simulink library "Lib_PF_SwitchDC_TMATS"  (R2017a)
settings: Solver=ode45  StartTime=0.0  StopTime=10.0  RelTol=1e-3  EnableMultiTasking=on
Description:
  | Thomas Modules
settings Model: Creator=jwchapm2  LastModifiedBy=glthoma1
settings DataIOCC: LimitDataPoints=on  SaveFormat=Array
settings OptimizationCC: ExpressionDepthLimit=2147483647  LifeSpan=inf
settings DebuggingCC: UnderspecifiedInitializationDetection=Classic  MergeDetectMultiDrivingBlocksExec=none  SolverPrmCheckMsg=warning  StateNameClashWarn=warning  SFUnexpectedBacktrackingDiag=warning  SFNoUnconditionalDefaultTransitionDiag=warning  SFExecutionAtInitializationDiag=none
settings HardwareCC: ProdBitPerPointer=32  ProdBitPerSizeT=32  ProdBitPerPtrDiffT=32  ProdLargestAtomicFloat=None  ProdIntDivRoundTo=Undefined  ProdEndianess=Unspecified  ProdWordSize=32  ProdHWDeviceType=32-bit Generic
settings ModelReferenceCC: PropagateSignalLabelsOutOfModel=off
settings GRTTargetCC: TargetLangStandard=C89/C90 (ANSI)  GeneratePreprocessorConditionals=Disable all
settings ConfigComp: CovMetricSettings=dw  CovHtmlReporting=on  CovSaveCumulativeToWorkspaceVar=on  CovSaveSingleToWorkspaceVar=on  CovExternalEMLEnable=off

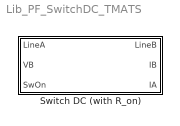
== system Lib_PF_SwitchDC_TMATS ==
  Switch DC (with R_on) : Subsystem  mask{R_M=100}
      mask prompts: R_M "R_M - On Resistance"
      mask Display:
      | fprintf('R_on: %g',R_M)
      | port_label('input',1,'VA')
      | port_label('input',2,'VBg')
      | port_label('input',3,'SwOn')
      | port_label('output',1,'VB')
      | port_label('output',2,'IB')
      | port_label('output',3,'IA')

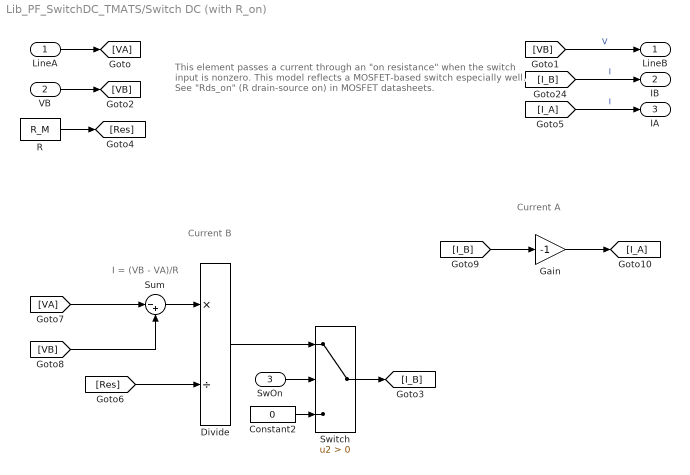
== system Lib_PF_SwitchDC_TMATS/Switch DC (with R_on) ==
  note: This element passes a current through an "on resistance"
      | when the switch input is nonzero.
      | This model reflects a MOSFET-based switch especially well.
      | See "Rds_on" (R drain-source on) in MOSFET datasheets.
  note: I = (VB - VA)/R
  note: Current B
  note: Current A
  LineA : Inport
  VB : Inport  Port=2
  SwOn : Inport  Port=3
  Constant2 : Constant  Value=0
  Divide : Product  Inputs=*/
  Gain : Gain  Gain=-1
  R : Constant  Value=R_M
  Sum : Sum  Inputs=|-+
  Switch : Switch  Criteria=u2 > Threshold
  LineB : Outport
  IB : Outport  Port=2
  IA : Outport  Port=3
  wires:
  LineA/1 -> [VA]
  [I_A] -> IA/1  "I"
  VB/1 -> [VB]
  [VB] -> LineB/1  "V"
  R/1 -> [Res]
  [I_B] -> IB/1  "I"
  [VB] -> Sum/2
  [VA] -> Sum/1
  Divide/1 -> Switch/1
  Sum/1 -> Divide/1
  [Res] -> Divide/2
  [I_B] -> Gain/1
  Gain/1 -> [I_A]
  SwOn/1 -> Switch/2
  Switch/1 -> [I_B]
  Constant2/1 -> Switch/3
